simulink model "BatteryController_Rev1"  (Simulink 7.7)
settings: Solver=FixedStepDiscrete  StartTime=0.0  StopTime=10.0  RelTol=1e-3
PreLoadFcn:
  | try, eval([bdroot '_setup']); catch, eval('model_setup', ''); end
InitFcn:
  | try, eval([bdroot '_setup']); catch, eval('model_setup', ''); end
undefined symbols (not defined in the file or in its folder): ECU555, motohawk_build_version, motohawk_trunc_name, motohawk_vardec_path
libraries: MotoHawk_lib x213, motohawk_annotations_lib x6, motohawk_control_primitives_lib x2, simulink x1
(part 1 of 4)
Description:
  | Template Project Model
CloseFcn:
  | try, eval([bdroot '_close']); catch, eval('model_close', ''); end
settings Model: MotoHawkBuildVersion=073  MotoHawkBuildStats=struct('TotalFLASH',{0},'TotalEEPROM',{0},'TotalRAM',{0},'AppFLASH',{0},'AppEEPROM',{0},'AppRAM',{0},'HeapRAM',{0},'BuildSuccessCount',{73},'BuildErrorCount',{2})  MotoHawkModelSavedName=BatteryController_Rev1  MotoHawkModelGUID=1c823790-94c1-4f9f-95-ed-5c-78-f7-df-2e  MotoHawkModelOpenTime=2018 8 25 20 24 10.197  MotoHawkModelElapsedTime=15675530.773  MotoHawkBuildInfo=struct('model_name',{'BatteryController_Rev1'},'motohawk_version',{'2011a_sp0.184'},'motohawk_component_version',{'0.0.7'},'matlab_version',{'7.12.0'},'build_version',{'072'},'module_type',{'ECU555-48-0707'},'layout_type',{'PROD'},'processor_family',{'PPC'},'processor_type',{'MPC555'},'toolchain_vendor',{'gcc-powerpc-eabi'},'toolchain_version',{'4.4.0'},'component',{0},'archive_file',{'ECM.a'},'enable_build',{1},'fptype',{0},'flash_size',{368640},'ee_size',{4096},'ram_size',{26624},'decram_size',{0},'module_memory_def',{'MPC555_ModMemoryDef_4KEE_Prod'},'eri_table0_rev',{9},'max_eri_table_size',{65535},'use_debug_vardecs',{1},'use_info_vardecs',{1},'fgnd_base_period_ms',{5},'bgnd_base_period_ms',{50},'root_build_dir',{'C:\Users\maxar\Documents\GitHub\Wisconsin-Hybrid\BatteryController_Rev1'},'build_dir',{'C:\Users\maxar\Documents\GitHub\Wisconsin-Hybrid\BatteryController_Rev1\BatteryController_Rev1_Build'},'dll_name',{'BatteryCo_072'},'srz_name',{'BatteryController_Rev1_072'},'fgnd_stack_size',{3072},'fgnd_angle_stack_size',{0},'bgnd_stack_size',{2048},'idle_stack_size',{1024},'irq_stack_size',{1536},'heap_size',{4096},'heap_margin',{409},'install_dll_dir',{'C:\ECUFiles\TDBDLL\'},'install_srz_dir',{'C:\ECUFiles\Programs'},'app_int_stack_size',{1024},'shutdown_stack_size',{1024},'mingw_dir',{'C:\PROGRA~2\Woodward\DEVELO~1\TOOLCH~1\GCC\win32-pe\4_4_0\'},'motohawk_dir',{'C:\PROGRA~2\Woodward\MCS\MotoHawk\2011A_~1.184'},'toolchain_dir',{'C:\Program Files (x86)\Woodward\DevelopmentTools\Toolchains\GCC\powerpc-eabi\4_4_0\'},'matlab_root',{'C:\Program Files (x86)\MATLAB\R2011a'},'model_guid',{'1c823790-94c1-4f9f-95-ed-5c-78-f7-df-2e'},'build_guid',{'2c20b1f2-2f68-4f6b-8e-8e-5f-43-f8-60-40'},'token_guid',{'DD8AD11F95A6FC42BFF9AC780840E4B4'})  MotoHawkBuildGUID=2c20b1f2-2f68-4f6b-8e-8e-5f-43-f8-60-40  Creator=Owner  LastModifiedBy=maxar
settings OptimizationCC: InlineParams=on  InitFltsAndDblsToZero=on  OptimizeModelRefInitCode=on  LifeSpan=1
settings DebuggingCC: SolverPrmCheckMsg=none  InheritedTsInSrcMsg=none  TasksWithSamePriorityMsg=none  StrictBusMsg=Warning
settings HardwareCC: ProdEndianess=BigEndian  ProdHWDeviceType=Specified
settings RTWCC: SystemTargetFile=motohawk_ert_rtw.tlc  TLCOptions="-aCustomNonFinites=\"motohawk_genrtnonfinite.tlc\""  MakeCommand=motohawk_make_rtw  TemplateMakefile=motohawk_ert_rtw.tmf  Description=MotoHawk(tm) Rapid Prototyping  ProcessScript=motohawk_ert_rtw_make_rtw_hook
settings CodeAppCC: IgnoreCustomStorageClasses=off  MaxIdLength=100  CustomSymbolStrField=$H$N$M
settings STFCustomTargetCC: FunctionExecutionProfile=off  ModelReferenceCompliant=off  CombineOutputUpdateFcns=on  ERTCustomFileBanners=on  SupportContinuousTime=off  SupportNonInlinedSFcns=off  SystemTargetFile=motohawk_ert_rtw.tlc
settings ERTTargetCC: FunctionExecutionProfile=off  MultiwordLength=2048  ModelReferenceCompliant=off  ParMdlRefBuildCompliant=off  CompOptLevelCompliant=off  ERTFirstTimeCompliant=off  ModelStepFunctionPrototypeControlCompliant=off  CPPClassGenCompliant=off  ERTCustomFileTemplate=example_file_process.tlc  ConvertIfToSwitch=off

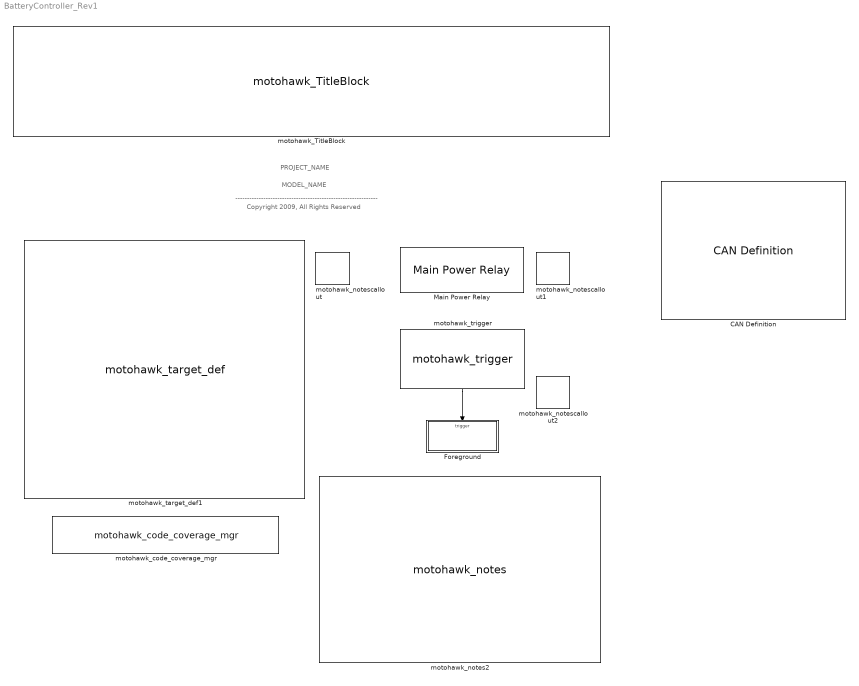
== system BatteryController_Rev1 ==
  note: PROJECT_NAME
  note: MODEL_NAME
  note: -------------------------------------------------------------
  note: Copyright 2009, All Rights Reserved
  CAN Definition : MotoHawk_lib/CAN Blocks/CAN Definition  Priority=-100  nam='CAN_1'  text_resource=CAN1  code_resource=NONE  val_resource=-1  target=ECU555-48-0707  bus=-2  btime=500 kbaud  pre=1  prop=0  pseg1=0  pseg2=0  resyn=0  tx_queue_size=16  rx_queue_size=16  use_protocol=on  city_id=hex2dec('D')  access_level=4  mototune_group='System | System Config | Communication Config'
  Foreground : Subsystem  TreatAsAtomicUnit=on
      mask init:
      | SampleTime = 0.005;
      | lbl = sprintf('%d ms', SampleTime * 1000);
      settings: RTWSystemCode=Function  RTWFcnNameOpts=Use subsystem name  RTWFileNameOpts=Use function name
      mask Display: disp(lbl);
  Main Power Relay : MotoHawk_lib/Extra Development Blocks/Main Power Relay  SystemSampleTime=-1  on_delay_count=2  off_delay_count=5  ecup_threshold=100  group='System | Main Power Relay'
  motohawk_TitleBlock : motohawk_annotations_lib/motohawk_TitleBlock  BlockType_='Mototron_Title_Block'  ttl="[  strrep(get_param(bdroot, 'Description') , '_', '\\_')  '\\newline\\rm'  'Top-level root of model:  '   strrep(bdroot, '_', '\\_') '.mdl'  ]"  copyright="'THE INFORMATION CONTAINED IN THIS\\newlineDRAWING IS THE SOLE PROPERTY OF\\newlineWOODWARD.  ANY REPRODUCTION IN\\newline PART OR AS A WHOLE WITHOUT THE\\newlineWRITTEN PERMISSION OF WOODWARD\\newline IS PROHIBITED.\\fontsize{16}\\rm\\copyright\\rm\\fontsize{10} 2009'"  address='\fontsize{22}\it\fontname{Arial Black}Woodward \fontname{Arial}\fontsize{10}\newline1000 East Drake Road, Fort Collins, CO, 80525\newlinemcs.woodward.com (866) 588-0494'  image_file='mh.jpg'  pretty_print=on  edit_text=|  edit_as=5
      | [
      | 
      | 
      | 
      | 
      | 
      | strrep(get_param(bdroot, 'Description') , '_', '\_')  '\newline\rm'
      | 
      | 
      | 
      | 
      | 
      | 'Top-level root of model:  '   strrep(bdroot, '_', '\_') '.mdl'
      | 
      | 
      | 
      | 
      | 
      | ]
  motohawk_code_coverage_mgr : MotoHawk_lib/Extra Development Blocks/motohawk_code_coverage_mgr  codegen=Always Generate Code Coverage Code  group='System | Code Coverage'
  motohawk_notes2 : motohawk_annotations_lib/motohawk_notes  BlockType_='Mototron_Notes'  desc="'\\fontname{wingdings 2}u\\fontname{arial}  The existence of a Target Definition block\\newlinesomewhere in the model sets it up as a\\newlineMotoHawk project, capable of being built to a\\newlineMotoTron target module.\\newline\\newline\\fontname{wingdings 2}v\\fontname{arial}  The Main Power Relay block monitors the\\newlinemodule power and controls the Main Power Relay\\newlineIt also performs startup and shutdown procedures\\newlinenecessary for EEPROM storage.  Most designs\\newlineshould contain this block\\newline\\newline\\fontname{wingdings 2}w\\fontname{arial}  All actions must be performed inside of a\\newlinefunction-call subsystem, triggered by a MotoHawk\\newlineentry-point trigger block, in order to be included in the\\newlinegenerated code.\\newline'"  edit_text=|  edit_as=2
      | \fontname{wingdings 2}u\fontname{arial}  The existence of a Target Definition block
      | 
      | 
      | somewhere in the model sets it up as a
      | 
      | 
      | MotoHawk project, capable of being built to a
      | 
      | 
      | Woodward target module.
      | 
      | 
      | 
      | 
      | 
      | \fontname{wingdings 2}v\fontname{arial}  The Main Power Relay block monitors the
      | 
      | 
      | module power and controls the Main Power Relay
      | 
      | 
      | It also performs startup and shutdown procedures
      | 
      | 
      | necessary for EEPROM storage.  Most designs
      | 
      | 
      | should contain this block
      | 
      | 
      | 
      | 
      | 
      | \fontname{wingdings 2}w\fontname{arial}  All actions must be performed inside of a
      | 
      | 
      | function-call subsystem, triggered by a MotoHawk
      | 
      | 
      | entry-point trigger block, in order to be included in the
      | 
      | 
      | generated code.
  motohawk_notescallout : motohawk_annotations_lib/motohawk_notescallout  BlockType_='Mototron_NoteCall'  desc='\bf1'
  motohawk_notescallout1 : motohawk_annotations_lib/motohawk_notescallout  BlockType_='Mototron_NoteCall'  desc='\bf2'
  motohawk_notescallout2 : motohawk_annotations_lib/motohawk_notescallout  BlockType_='Mototron_NoteCall'  desc='\bf3'
  motohawk_target_def1 : MotoHawk_lib/motohawk_target_def  Priority=-65535  target=ECU555-48-0707  layout=PROD  fptype=single (32 bits)  fgnd_stack_size=3*1024  fgnd_angle_stack_size=0  bgnd_stack_size=2*1024  idle_stack_size=1024  irq_stack_size=1536  app_int_stack_size=1024  shutdown_stack_size=1024  heap_size=4*1024  show_margins=off  fgnd_stack_margin=(3*1024) * 0.1  fgnd_angle_stack_margin=0  bgnd_stack_margin=(2*1024) * 0.1  idle_stack_margin=(1024) * 0.1  irq_stack_margin=(1536) * 0.1  app_int_stack_margin=(1024) * 0.1  shutdown_stack_margin=(1024) * 0.1  heap_margin=(4*1024) * 0.1  comp_name=bdroot  comp_img='KVASER_CAN_USB.jpg'  comp_security=No Encryption  comp_build_pass='mhbuild'  comp_sim_pass='mhsim'  comp_multi=off  show_filenames=off  dll_name=motohawk_trunc_name(bdroot, ['_' motohawk_build_version], 13)  srz_name=motohawk_trunc_name(bdroot, ['_' motohawk_build_version], 50)  build_dir='.'  comp_dir='.'
  motohawk_trigger : MotoHawk_lib/Trigger Blocks/motohawk_trigger  Tag=Trigger  Priority=0  trigger=FGND_RTI_PERIODIC  function_name=Trigger_FGND_RTI_PERIODIC_1023p0001  priority_order=0  inherited=off  run_disabled=off  override_app_monitor=off  target=ECU555_48_0707
  wires:
  motohawk_trigger/1 -> Foreground/Trigger

== system BatteryController_Rev1/Foreground ==
  f : TriggerPort  TriggerType=function-call
  Battery : Subsystem
  motohawk_TitleBlock : motohawk_annotations_lib/motohawk_TitleBlock  BlockType_='Mototron_Title_Block'  ttl=[strrep(get_param(bdroot, 'Description') , '_', '\_') '\newline\rm' get_param(gcs, 'Name')]  copyright="'THE INFORMATION CONTAINED IN THIS\\newlineDRAWING IS THE SOLE PROPERTY OF\\newlineWOODWARD.  ANY REPRODUCTION IN\\newline PART OR AS A WHOLE WITHOUT THE\\newlineWRITTEN PERMISSION OF WOODWARD\\newline IS PROHIBITED.\\fontsize{16}\\rm\\copyright\\rm\\fontsize{10} 2009'"  address='\fontsize{22}\it\fontname{Arial Black}Woodward \fontname{Arial}\fontsize{10}\newline1000 East Drake Road, Fort Collins, CO, 80525\newlinemcs.woodward.com (866) 588-0494'  image_file='mh.jpg'  pretty_print=on  edit_text=[strrep(get_param(bdroot, 'Description') , '_', '\_') '\newline\rm' get_param(gcs, 'Name')]  edit_as=5
  motohawk_code_coverage : MotoHawk_lib/Extra Development Blocks/motohawk_code_coverage

== system BatteryController_Rev1/Foreground/Battery ==
  Control : Subsystem
  Inputs : Subsystem
  Outputs : Subsystem
  wires:
  Control/1(Out1) -> Outputs/2(Controlled Inputs)
  Inputs/1(Out1) -> Control/1(In1), Outputs/1(Inputs)

== system BatteryController_Rev1/Foreground/Battery/Control ==
  In1 : Inport
  AMP Clamp : Subsystem
  Battery States : Subsystem
  Bus Creator : BusCreator  Inputs=3
  SOC : Subsystem
  Out1 : Outport
  wires:
  In1/1 -> Battery States/1(In1), SOC/1(In1), AMP Clamp/1(In1)
  Bus Creator/1 -> Out1/1
  Battery States/1(Out1) -> Bus Creator/1  "Battery States"
  AMP Clamp/1(Out1) -> Bus Creator/2, SOC/2(Current), Battery States/2(Current)  "AMP Clamp"
  SOC/1(Out1) -> Bus Creator/3  "SOC"

== system BatteryController_Rev1/Foreground/Battery/Inputs ==
  2G BMS : Subsystem
  AMP Clamp : Subsystem
  Bus Creator : BusCreator  Inputs=3
  Contactors : Subsystem
  Out1 : Outport
  wires:
  Bus Creator/1 -> Out1/1
  Contactors/1(Out1) -> Bus Creator/1  "Contactors"
  2G BMS/1(Out1) -> Bus Creator/2  "2G BMS"
  AMP Clamp/1(Out1) -> Bus Creator/3  "AMP Clamp"

== system BatteryController_Rev1/Foreground/Battery/Outputs ==
  Inputs : Inport
  Controlled Inputs : Inport  Port=2
  Battery : Subsystem
  Contactors : Subsystem
  wires:
  Controlled Inputs/1 -> Contactors/1(In1), Battery/2(Controlled Inputs)
  Inputs/1 -> Contactors/2(In2), Battery/1(Inputs)

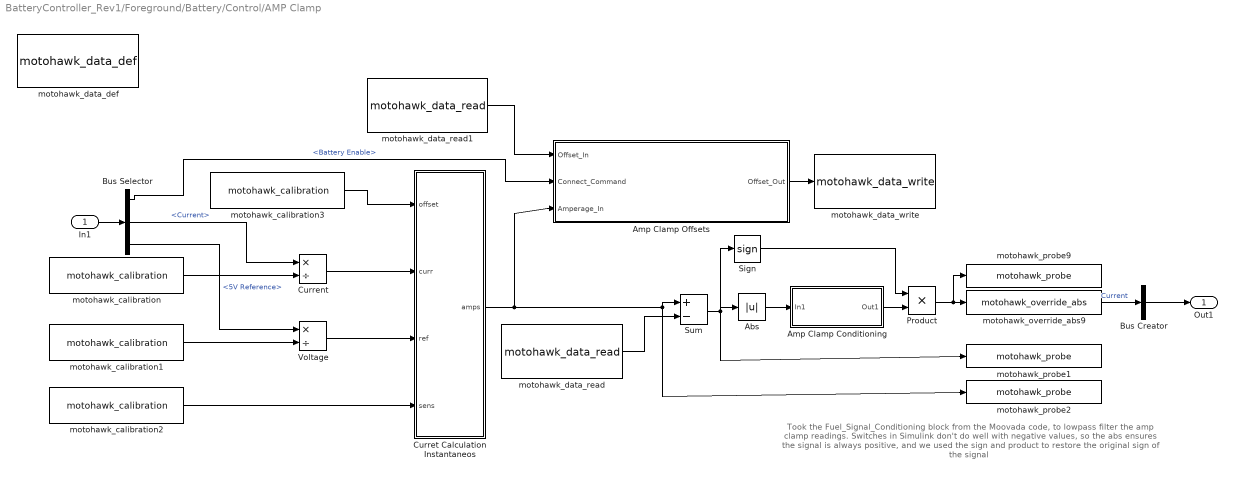
== system BatteryController_Rev1/Foreground/Battery/Control/AMP Clamp ==
  note: Took the Fuel_Signal_Conditioning block from the Moovada code, to lowpass filter the amp clamp readings.
      | Switches in Simulink don't do well with negative values, so the abs ensures the signal is always positive,
      | and we used the sign and product to restore the original sign of the signal
  In1 : Inport
  Abs : Abs
  Amp Clamp Conditioning : Subsystem
  Amp Clamp Offsets : Stateflow chart  TreatAsAtomicUnit=on
  Bus Creator : BusCreator  Inputs=1
  Bus Selector : BusSelector  OutputSignals=Contactors.Battery Enable,AMP Clamp.Current,AMP Clamp.5V Reference
  Current : Product  Inputs=*/  RndMeth=Zero
  Curret Calculation Instantaneos : Stateflow chart  TreatAsAtomicUnit=on
  Product : Product  RndMeth=Zero
  Sign : Signum
  Sum : Sum  Inputs=+-
  Voltage : Product  Inputs=*/  RndMeth=Zero
  motohawk_calibration : MotoHawk_lib/Calibration & Probing Blocks/motohawk_calibration  nam='Current_Div2'  val=819.2  storage=Calibration NV  show_more=off  name_source=Use Parameter  data_type=Inherit from 'Default Value'  read_level=1  write_level=1  ovr_cals=on  view_as=Number  enum_struct={'Disabled', 'Enabled'}  vector_style=Wide Row  use_help_units=off  help=''  units=''  use_header_enum=off  row_header_enum={}  col_header_enum={}  use_min_max=off  min_val=-inf  max_val=inf  use_precision=off  precision=''  gain=1  offset=0  exp=1  use_mototune_group=off  mototune_group=motohawk_vardec_path(gcb)
  motohawk_calibration1 : MotoHawk_lib/Calibration & Probing Blocks/motohawk_calibration  nam='V5V_Ref2'  val=409.6  storage=Calibration NV  show_more=off  name_source=Use Parameter  data_type=Inherit from 'Default Value'  read_level=1  write_level=1  ovr_cals=on  view_as=Number  enum_struct={'Disabled', 'Enabled'}  vector_style=Wide Row  use_help_units=off  help=''  units=''  use_header_enum=off  row_header_enum={}  col_header_enum={}  use_min_max=off  min_val=-inf  max_val=inf  use_precision=off  precision=''  gain=1  offset=0  exp=1  use_mototune_group=off  mototune_group=motohawk_vardec_path(gcb)
  motohawk_calibration2 : MotoHawk_lib/Calibration & Probing Blocks/motohawk_calibration  nam='G_Sensativity'  val=0.00615  storage=Calibration NV  show_more=on  name_source=Use Parameter  data_type=Inherit from 'Default Value'  read_level=1  write_level=1  ovr_cals=on  view_as=Number  enum_struct={'Disabled', 'Enabled'}  vector_style=Wide Row  use_help_units=on  help=''  units='V'  use_header_enum=off  row_header_enum={}  col_header_enum={}  use_min_max=off  min_val=-inf  max_val=inf  use_precision=on  precision='1.5'  gain=1  offset=0  exp=1  use_mototune_group=off  mototune_group=motohawk_vardec_path(gcb)
  motohawk_calibration3 : MotoHawk_lib/Calibration & Probing Blocks/motohawk_calibration  nam='AmpV_Offset'  val=2.15  storage=Calibration  show_more=off  name_source=Use Parameter  data_type=Inherit from 'Default Value'  read_level=1  write_level=1  ovr_cals=on  view_as=Number  enum_struct={'Disabled', 'Enabled'}  vector_style=Wide Row  use_help_units=off  help=''  units=''  use_header_enum=off  row_header_enum={}  col_header_enum={}  use_min_max=off  min_val=-inf  max_val=inf  use_precision=off  precision=''  gain=1  offset=0  exp=1  use_mototune_group=off  mototune_group=motohawk_vardec_path(gcb)
  motohawk_data_def : MotoHawk_lib/Data Storage Blocks/motohawk_data_def  nam='Amp_Offset'  container_nam=''  data=2.15  typ=double  struct_nam='MyStruct'  storage=NonVolatile  outputRef=off  use_vardec=on  window=Calibration  read_level=1  write_level=1  ovr_cals=on  view_as=Number  enum_struct={'Disabled', 'Enabled'}  vector_style=Wide Row  use_help_units=off  help=''  units=''  use_header_enum=off  row_header_enum=''  col_header_enum=''  use_min_max=off  min_val=-inf  max_val=inf  use_precision=off  precision=''  gain=1  offset=0  exp=1  use_mototune_group=off  mototune_group=motohawk_vardec_path(gcb)  eval_name=MyData  data_stores=motohawk_sfun_data_def_data_stores  struct_instances=motohawk_sfun_data_def_struct_instances  vardecs=motohawk_sfun_data_def_vardecs
  motohawk_data_read : MotoHawk_lib/Data Storage Blocks/motohawk_data_read  source=Lookup By Name  structure=Scalar  operation=Read scalar from location by index  sz_vec=4  sz_row=2  sz_col=3  typ=double  nam='Amp_Offset'  checkNull=on  struct_inst_name='MyData'  struct_nam='MyStruct'
  motohawk_data_read1 : MotoHawk_lib/Data Storage Blocks/motohawk_data_read  source=Lookup By Name  structure=Scalar  operation=Read scalar from location by index  sz_vec=4  sz_row=2  sz_col=3  typ=double  nam='Amp_Offset'  checkNull=on  struct_inst_name='MyData'  struct_nam='MyStruct'
  motohawk_data_write : MotoHawk_lib/Data Storage Blocks/motohawk_data_write  source=Lookup By Name  structure=Scalar  operation=Write entire data structure at once  sz_vec=9  sz_row=2  sz_col=9  typ=double  nam='Amp_Offset'  checkNull=on  write_read_only=off  struct_inst_name=''  struct_name='MyStruct'
  motohawk_override_abs9 : MotoHawk_lib/Calibration & Probing Blocks/motohawk_override_abs  SystemSampleTime=-1  parent_name='AMPCurrent_Ovr'  parent_val=0  show_more=on  name_source=Use Parameter  parent_read_level=1  parent_override_level=1  view_as=Number  enum_struct={'Disabled', 'Enabled'}  use_help_units=off  parent_help=''  parent_units=''  use_min_max=off  parent_min=-inf  parent_max=inf  use_precision=off  parent_precision=''  parent_gain=1  parent_offset=0  parent_exp=1  use_mototune_group=off  parent_group=motohawk_vardec_path(gcb)
  motohawk_probe1 : MotoHawk_lib/Calibration & Probing Blocks/motohawk_probe  nam='AMPCurrent_Pre_Filter_Prb'  show_more=on  name_source=Use Parameter  read_level=1  view_as=Number  enum_struct={'Disabled', 'Enabled'}  vector_style=Wide Row  use_help_units=on  help=''  units='A'  use_header_enum=off  row_header_enum={}  col_header_enum={}  use_precision=on  precision='1.5'  gain=1  offset=0  exp=1  use_mototune_group=off  mototune_group=motohawk_vardec_path(gcb)
  motohawk_probe2 : MotoHawk_lib/Calibration & Probing Blocks/motohawk_probe  nam='AMPCurrent_Pre_Offset_Prb'  show_more=on  name_source=Use Parameter  read_level=1  view_as=Number  enum_struct={'Disabled', 'Enabled'}  vector_style=Wide Row  use_help_units=on  help=''  units='A'  use_header_enum=off  row_header_enum={}  col_header_enum={}  use_precision=on  precision='1.5'  gain=1  offset=0  exp=1  use_mototune_group=off  mototune_group=motohawk_vardec_path(gcb)
  motohawk_probe9 : MotoHawk_lib/Calibration & Probing Blocks/motohawk_probe  nam='AMPCurrent_Prb'  show_more=on  name_source=Use Parameter  read_level=1  view_as=Number  enum_struct={'Disabled', 'Enabled'}  vector_style=Wide Row  use_help_units=on  help=''  units='A'  use_header_enum=off  row_header_enum={}  col_header_enum={}  use_precision=on  precision='1.5'  gain=1  offset=0  exp=1  use_mototune_group=off  mototune_group=motohawk_vardec_path(gcb)
  Out1 : Outport
  wires:
  In1/1 -> Bus Selector/1
  Bus Selector/2 -> Current/1  "<Current>"
  Bus Selector/3 -> Voltage/1  "<5V Reference>"
  Bus Creator/1 -> Out1/1
  motohawk_override_abs9/1 -> Bus Creator/1  "Current"
  motohawk_calibration1/1 -> Voltage/2
  motohawk_calibration/1 -> Current/2
  Current/1 -> Curret Calculation Instantaneos/2(curr)
  Voltage/1 -> Curret Calculation Instantaneos/3(ref)
  motohawk_calibration2/1 -> Curret Calculation Instantaneos/4(sens)
  Amp Clamp Conditioning/1(Out1) -> Product/2
  Sign/1 -> Product/1
  Product/1 -> motohawk_override_abs9/1, motohawk_probe9/1
  motohawk_calibration3/1 -> Curret Calculation Instantaneos/1(offset)
  Curret Calculation Instantaneos/1(amps) -> Amp Clamp Offsets/3(Amperage_In), Sum/1, motohawk_probe2/1
  Amp Clamp Offsets/1(Offset_Out) -> motohawk_data_write/1
  motohawk_data_read/1 -> Sum/2
  Sum/1 -> Abs/1, Sign/1, motohawk_probe1/1
  Abs/1 -> Amp Clamp Conditioning/1(In1)
  Bus Selector/1 -> Amp Clamp Offsets/2(Connect_Command)  "<Battery Enable>"
  motohawk_data_read1/1 -> Amp Clamp Offsets/1(Offset_In)

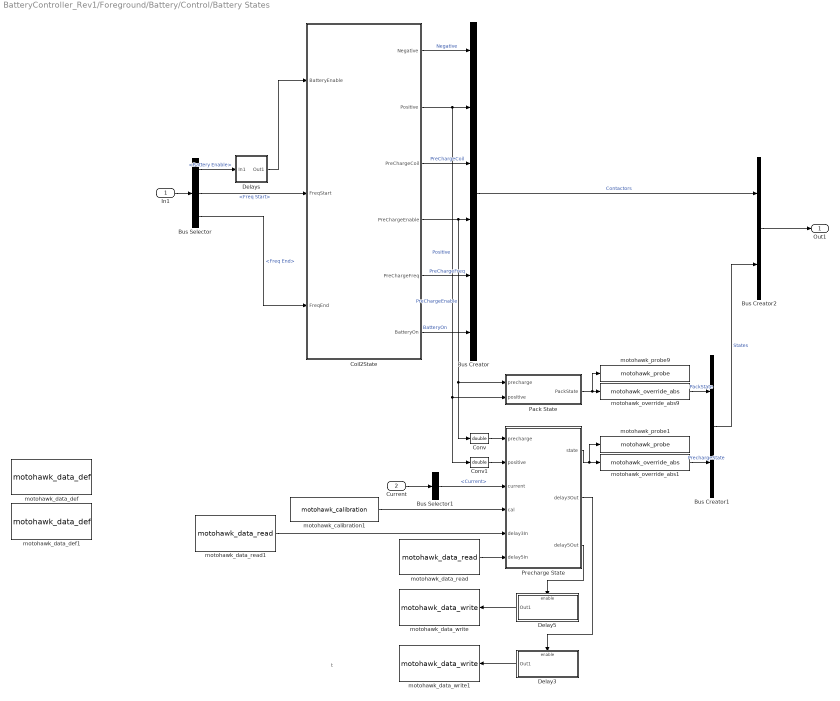
== system BatteryController_Rev1/Foreground/Battery/Control/Battery States ==
  note: t
  In1 : Inport
  Current : Inport  Port=2
  Bus Creator : BusCreator  Inputs=6
  Bus Creator1 : BusCreator  Inputs=2
  Bus Creator2 : BusCreator  Inputs=2
  Bus Selector : BusSelector  OutputSignals=Contactors.Battery Enable,Contactors.Freq Start,Contactors.Freq End
  Bus Selector1 : BusSelector  OutputSignals=Current
  Coil2State : Stateflow chart  TreatAsAtomicUnit=on
  Conv : DataTypeConversion  OutDataTypeStr=double
  Conv1 : DataTypeConversion  OutDataTypeStr=double
  Delay3 : Subsystem  TreatAsAtomicUnit=on
  Delay5 : Subsystem  TreatAsAtomicUnit=on
  Delays : Subsystem
  Pack State : Stateflow chart  TreatAsAtomicUnit=on
  Precharge State : Stateflow chart  TreatAsAtomicUnit=on
  motohawk_calibration1 : MotoHawk_lib/Calibration & Probing Blocks/motohawk_calibration  nam='Precharge_Current_Threshold'  val=.75  storage=Calibration NV  show_more=on  name_source=Use Parameter  data_type=Inherit from 'Default Value'  read_level=1  write_level=1  ovr_cals=on  view_as=Number  enum_struct={'Disabled', 'Enabled'}  vector_style=Wide Row  use_help_units=off  help=''  units=''  use_header_enum=off  row_header_enum={}  col_header_enum={}  use_min_max=off  min_val=-inf  max_val=inf  use_precision=off  precision=''  gain=1  offset=0  exp=1  use_mototune_group=off  mototune_group=motohawk_vardec_path(gcb)
  motohawk_data_def : MotoHawk_lib/Data Storage Blocks/motohawk_data_def  nam='Delay5'  container_nam=''  data=0  typ=boolean  struct_nam='MyStruct'  storage=Volatile  outputRef=off  use_vardec=on  window=Calibration  read_level=1  write_level=1  ovr_cals=on  view_as=Number  enum_struct={'Disabled', 'Enabled'}  vector_style=Wide Row  use_help_units=off  help=''  units=''  use_header_enum=off  row_header_enum=''  col_header_enum=''  use_min_max=off  min_val=-inf  max_val=inf  use_precision=off  precision=''  gain=1  offset=0  exp=1  use_mototune_group=off  mototune_group=motohawk_vardec_path(gcb)  eval_name=MyData  data_stores=motohawk_sfun_data_def_data_stores  struct_instances=motohawk_sfun_data_def_struct_instances  vardecs=motohawk_sfun_data_def_vardecs
  motohawk_data_def1 : MotoHawk_lib/Data Storage Blocks/motohawk_data_def  nam='Delay3'  container_nam=''  data=0  typ=boolean  struct_nam='MyStruct'  storage=Volatile  outputRef=off  use_vardec=on  window=Calibration  read_level=1  write_level=1  ovr_cals=on  view_as=Number  enum_struct={'Disabled', 'Enabled'}  vector_style=Wide Row  use_help_units=off  help=''  units=''  use_header_enum=off  row_header_enum=''  col_header_enum=''  use_min_max=off  min_val=-inf  max_val=inf  use_precision=off  precision=''  gain=1  offset=0  exp=1  use_mototune_group=off  mototune_group=motohawk_vardec_path(gcb)  eval_name=MyData  data_stores=motohawk_sfun_data_def_data_stores  struct_instances=motohawk_sfun_data_def_struct_instances  vardecs=motohawk_sfun_data_def_vardecs
  motohawk_data_read : MotoHawk_lib/Data Storage Blocks/motohawk_data_read  source=Lookup By Name  structure=Scalar  operation=Read scalar from location by index  sz_vec=4  sz_row=2  sz_col=3  typ=boolean  nam='Delay5'  checkNull=on  struct_inst_name='MyData'  struct_nam='MyStruct'
  motohawk_data_read1 : MotoHawk_lib/Data Storage Blocks/motohawk_data_read  source=Lookup By Name  structure=Scalar  operation=Read scalar from location by index  sz_vec=4  sz_row=2  sz_col=3  typ=boolean  nam='Delay3'  checkNull=on  struct_inst_name='MyData'  struct_nam='MyStruct'
  motohawk_data_write : MotoHawk_lib/Data Storage Blocks/motohawk_data_write  source=Lookup By Name  structure=Scalar  operation=Write entire data structure at once  sz_vec=9  sz_row=2  sz_col=9  typ=boolean  nam='Delay5'  checkNull=on  write_read_only=off  struct_inst_name=''  struct_name='MyStruct'
  motohawk_data_write1 : MotoHawk_lib/Data Storage Blocks/motohawk_data_write  source=Lookup By Name  structure=Scalar  operation=Write entire data structure at once  sz_vec=9  sz_row=2  sz_col=9  typ=boolean  nam='Delay3'  checkNull=on  write_read_only=off  struct_inst_name=''  struct_name='MyStruct'
  motohawk_override_abs1 : MotoHawk_lib/Calibration & Probing Blocks/motohawk_override_abs  SystemSampleTime=-1  parent_name='PrechargeState__Ovr'  parent_val=0  show_more=on  name_source=Use Parameter  parent_read_level=1  parent_override_level=1  view_as=Number  enum_struct={'Disabled', 'Enabled'}  use_help_units=off  parent_help=''  parent_units=''  use_min_max=off  parent_min=-inf  parent_max=inf  use_precision=off  parent_precision=''  parent_gain=1  parent_offset=0  parent_exp=1  use_mototune_group=off  parent_group=motohawk_vardec_path(gcb)
  motohawk_override_abs9 : MotoHawk_lib/Calibration & Probing Blocks/motohawk_override_abs  SystemSampleTime=-1  parent_name='PackState__Ovr'  parent_val=0  show_more=on  name_source=Use Parameter  parent_read_level=1  parent_override_level=1  view_as=Number  enum_struct={'Disabled', 'Enabled'}  use_help_units=off  parent_help=''  parent_units=''  use_min_max=off  parent_min=-inf  parent_max=inf  use_precision=off  parent_precision=''  parent_gain=1  parent_offset=0  parent_exp=1  use_mototune_group=off  parent_group=motohawk_vardec_path(gcb)
  motohawk_probe1 : MotoHawk_lib/Calibration & Probing Blocks/motohawk_probe  nam='PreChargeState__Prb'  show_more=on  name_source=Use Parameter  read_level=1  view_as=Number  enum_struct={'Disabled', 'Enabled'}  vector_style=Wide Row  use_help_units=off  help=''  units=''  use_header_enum=off  row_header_enum={}  col_header_enum={}  use_precision=off  precision=''  gain=1  offset=0  exp=1  use_mototune_group=off  mototune_group=motohawk_vardec_path(gcb)
  motohawk_probe9 : MotoHawk_lib/Calibration & Probing Blocks/motohawk_probe  nam='PackState__Prb'  show_more=on  name_source=Use Parameter  read_level=1  view_as=Number  enum_struct={'Disabled', 'Enabled'}  vector_style=Wide Row  use_help_units=off  help=''  units=''  use_header_enum=off  row_header_enum={}  col_header_enum={}  use_precision=off  precision=''  gain=1  offset=0  exp=1  use_mototune_group=off  mototune_group=motohawk_vardec_path(gcb)
  Out1 : Outport
  wires:
  In1/1 -> Bus Selector/1
  Bus Selector/2 -> Coil2State/2(FreqStart)  "<Freq Start>"
  Bus Selector/3 -> Coil2State/3(FreqEnd)  "<Freq End>"
  Coil2State/1(Negative) -> Bus Creator/1  "Negative"
  Coil2State/2(Positive) -> Bus Creator/2, Pack State/2(positive), Conv1/1  "Positive"
  Coil2State/3(PreChargeCoil) -> Bus Creator/3  "PreChargeCoil"
  Coil2State/4(PreChargeEnable) -> Bus Creator/4, Pack State/1(precharge), Conv/1  "PreChargeEnable"
  Coil2State/5(PreChargeFreq) -> Bus Creator/5  "PreChargeFreq"
  Coil2State/6(BatteryOn) -> Bus Creator/6  "BatteryOn"
  Current/1 -> Bus Selector1/1
  Bus Selector1/1 -> Precharge State/3(current)  "<Current>"
  motohawk_calibration1/1 -> Precharge State/4(cal)
  Bus Creator/1 -> Bus Creator2/1  "Contactors"
  Bus Creator2/1 -> Out1/1
  Bus Creator1/1 -> Bus Creator2/2  "States"
  Pack State/1(PackState) -> motohawk_override_abs9/1, motohawk_probe9/1
  motohawk_override_abs9/1 -> Bus Creator1/1  "PackState"
  Precharge State/1(state) -> motohawk_override_abs1/1, motohawk_probe1/1
  motohawk_override_abs1/1 -> Bus Creator1/2  "PrechargeState"
  Conv/1 -> Precharge State/1(precharge)
  Conv1/1 -> Precharge State/2(positive)
  Precharge State/2(delay3Out) -> Delay3/Enable
  Precharge State/3(delay5Out) -> Delay5/Enable
  motohawk_data_read/1 -> Precharge State/6(delay5In)
  Delay5/1(Out1) -> motohawk_data_write/1
  motohawk_data_read1/1 -> Precharge State/5(delay3In)
  Delay3/1(Out1) -> motohawk_data_write1/1
  Bus Selector/1 -> Delays/1(In1)  "<Battery Enable>"
  Delays/1(Out1) -> Coil2State/1(BatteryEnable)

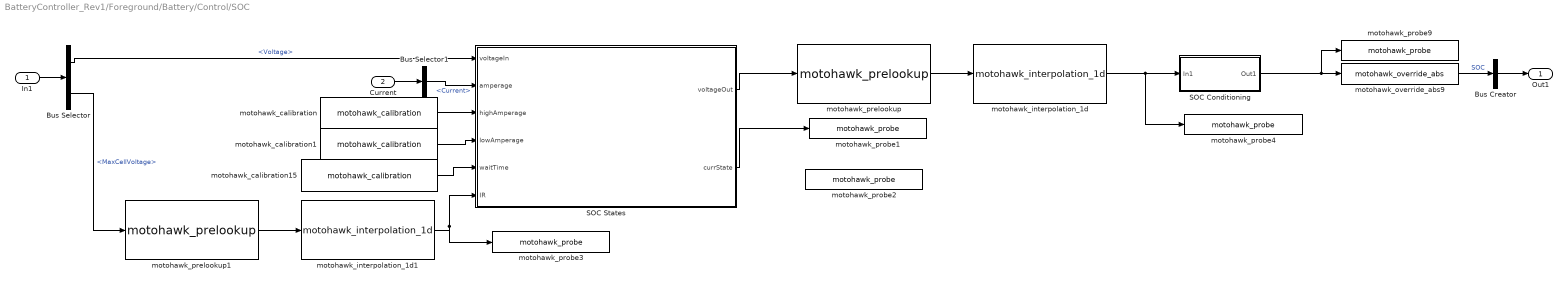
== system BatteryController_Rev1/Foreground/Battery/Control/SOC ==
  In1 : Inport
  Current : Inport  Port=2
  Bus Creator : BusCreator  Inputs=1
  Bus Selector : BusSelector  OutputSignals=2G BMS.Voltage,2G BMS.MaxCellVoltage
  Bus Selector1 : BusSelector  OutputSignals=Current
  SOC Conditioning : Subsystem
  SOC States : Stateflow chart  TreatAsAtomicUnit=on
  motohawk_calibration : MotoHawk_lib/Calibration & Probing Blocks/motohawk_calibration  nam='highAmperage'  val=25  storage=Calibration NV  show_more=on  name_source=Use Parameter  data_type=Inherit from 'Default Value'  read_level=1  write_level=1  ovr_cals=on  view_as=Number  enum_struct={'Disabled', 'Enabled'}  vector_style=Wide Row  use_help_units=off  help=''  units=''  use_header_enum=off  row_header_enum={}  col_header_enum={}  use_min_max=off  min_val=-inf  max_val=inf  use_precision=off  precision=''  gain=1  offset=0  exp=1  use_mototune_group=off  mototune_group=motohawk_vardec_path(gcb)
  motohawk_calibration1 : MotoHawk_lib/Calibration & Probing Blocks/motohawk_calibration  nam='lowAmperage'  val=20  storage=Calibration NV  show_more=on  name_source=Use Parameter  data_type=Inherit from 'Default Value'  read_level=1  write_level=1  ovr_cals=on  view_as=Number  enum_struct={'Disabled', 'Enabled'}  vector_style=Wide Row  use_help_units=on  help=''  units=''  use_header_enum=off  row_header_enum={}  col_header_enum={}  use_min_max=off  min_val=-inf  max_val=inf  use_precision=off  precision=''  gain=1  offset=0  exp=1  use_mototune_group=off  mototune_group=motohawk_vardec_path(gcb)
  motohawk_calibration15 : MotoHawk_lib/Calibration & Probing Blocks/motohawk_calibration  nam='Wait_time'  val=50  storage=Calibration NV  show_more=on  name_source=Use Parameter  data_type=int32  read_level=1  write_level=1  ovr_cals=on  view_as=Number  enum_struct={'Disabled', 'Enabled'}  vector_style=Wide Row  use_help_units=off  help=''  units=''  use_header_enum=off  row_header_enum={}  col_header_enum={}  use_min_max=off  min_val=-inf  max_val=inf  use_precision=on  precision=''  gain=0.05  offset=0  exp=1  use_mototune_group=off  mototune_group=motohawk_vardec_path(gcb)
  motohawk_interpolation_1d : MotoHawk_lib/Lookup Tables/motohawk_interpolation_1d  nam='SOCMap'  table_data=[100,99,8,0]  show_more=on  data_type=double  storage=Adaptive - NonVolatile  read_level=1  write_level=1  ovr_cals=on  use_help=off  help=''  units=''  use_min_max=on  min_val=0  max_val=100  use_precision=off  precision='1.2'  gain=1  offset=0  exp=1  use_links=on  prelookup_block='SOC_Table'  output_name=''  use_mototune_group=off  mototune_group=motohawk_vardec_path(gcb)
  motohawk_interpolation_1d1 : MotoHawk_lib/Lookup Tables/motohawk_interpolation_1d  nam='Temp_IR_Map'  table_data=[0.9,0.5,0.2,0.1,0.1]  show_more=on  data_type=double  storage=Adaptive - NonVolatile  read_level=1  write_level=1  ovr_cals=on  use_help=off  help=''  units=''  use_min_max=on  min_val=0  max_val=100  use_precision=off  precision='1.2'  gain=1  offset=0  exp=1  use_links=on  prelookup_block='Temp_IR_Table'  output_name=''  use_mototune_group=off  mototune_group=motohawk_vardec_path(gcb)
  motohawk_override_abs9 : MotoHawk_lib/Calibration & Probing Blocks/motohawk_override_abs  SystemSampleTime=-1  parent_name='SOC_Ovr'  parent_val=0  show_more=on  name_source=Use Parameter  parent_read_level=1  parent_override_level=1  view_as=Number  enum_struct={'Disabled', 'Enabled'}  use_help_units=off  parent_help=''  parent_units=''  use_min_max=off  parent_min=-inf  parent_max=inf  use_precision=off  parent_precision=''  parent_gain=1  parent_offset=0  parent_exp=1  use_mototune_group=off  parent_group=motohawk_vardec_path(gcb)
  motohawk_prelookup : MotoHawk_lib/Lookup Tables/motohawk_prelookup  nam='SOC_Table'  breakpoint_data=[385.95,378.51,319.92,279]  show_more=on  data_type=double  storage=NonVolatile  read_level=1  write_level=1  ovr_cals=on  use_help=off  help=''  units=''  use_min_max=off  min_val=-inf  max_val=inf  use_precision=off  precision=''  gain=1  offset=0  exp=1  use_links=off  input_name=''  use_mototune_group=off  mototune_group=motohawk_vardec_path(gcb)
  motohawk_prelookup1 : MotoHawk_lib/Lookup Tables/motohawk_prelookup  nam='Temp_IR_Table'  breakpoint_data=[-40,-20,0,20,40]  show_more=on  data_type=double  storage=NonVolatile  read_level=1  write_level=1  ovr_cals=on  use_help=off  help=''  units=''  use_min_max=off  min_val=-inf  max_val=inf  use_precision=off  precision=''  gain=1  offset=0  exp=1  use_links=off  input_name=''  use_mototune_group=off  mototune_group=motohawk_vardec_path(gcb)
  motohawk_probe1 : MotoHawk_lib/Calibration & Probing Blocks/motohawk_probe  nam='currState_Prb'  show_more=off  name_source=Use Parameter  read_level=1  view_as=Number  enum_struct={'Disabled', 'Enabled'}  vector_style=Wide Row  use_help_units=off  help=''  units=''  use_header_enum=off  row_header_enum={}  col_header_enum={}  use_precision=off  precision=''  gain=1  offset=0  exp=1  use_mototune_group=off  mototune_group=motohawk_vardec_path(gcb)
  motohawk_probe2 : MotoHawk_lib/Calibration & Probing Blocks/motohawk_probe  nam='vdiff_est_Prb'  show_more=off  name_source=Use Parameter  read_level=1  view_as=Number  enum_struct={'Disabled', 'Enabled'}  vector_style=Wide Row  use_help_units=off  help=''  units=''  use_header_enum=off  row_header_enum={}  col_header_enum={}  use_precision=off  precision=''  gain=1  offset=0  exp=1  use_mototune_group=off  mototune_group=motohawk_vardec_path(gcb)
  motohawk_probe3 : MotoHawk_lib/Calibration & Probing Blocks/motohawk_probe  nam='Temp_IR_Map_Prb'  show_more=off  name_source=Use Parameter  read_level=1  view_as=Number  enum_struct={'Disabled', 'Enabled'}  vector_style=Wide Row  use_help_units=off  help=''  units=''  use_header_enum=off  row_header_enum={}  col_header_enum={}  use_precision=off  precision=''  gain=1  offset=0  exp=1  use_mototune_group=off  mototune_group=motohawk_vardec_path(gcb)
  motohawk_probe4 : MotoHawk_lib/Calibration & Probing Blocks/motohawk_probe  nam='SOC_PreFilter_Prb'  show_more=off  name_source=Use Parameter  read_level=1  view_as=Number  enum_struct={'Disabled', 'Enabled'}  vector_style=Wide Row  use_help_units=off  help=''  units=''  use_header_enum=off  row_header_enum={}  col_header_enum={}  use_precision=off  precision=''  gain=1  offset=0  exp=1  use_mototune_group=off  mototune_group=motohawk_vardec_path(gcb)
  motohawk_probe9 : MotoHawk_lib/Calibration & Probing Blocks/motohawk_probe  nam='SOC_Prb'  show_more=on  name_source=Use Parameter  read_level=1  view_as=Number  enum_struct={'Disabled', 'Enabled'}  vector_style=Wide Row  use_help_units=off  help=''  units=''  use_header_enum=off  row_header_enum={}  col_header_enum={}  use_precision=off  precision=''  gain=1  offset=0  exp=1  use_mototune_group=off  mototune_group=motohawk_vardec_path(gcb)
  Out1 : Outport
  wires:
  In1/1 -> Bus Selector/1
  Bus Creator/1 -> Out1/1
  SOC States/1(voltageOut) -> motohawk_prelookup/1
  SOC States/2(currState) -> motohawk_probe1/1
  motohawk_calibration/1 -> SOC States/3(highAmperage)
  motohawk_calibration1/1 -> SOC States/4(lowAmperage)
  Current/1 -> Bus Selector1/1
  motohawk_override_abs9/1 -> Bus Creator/1  "SOC"
  motohawk_prelookup/1 -> motohawk_interpolation_1d/1
  motohawk_calibration15/1 -> SOC States/5(waitTime)
  ? -> motohawk_probe2/1
  Bus Selector/1 -> SOC States/1(voltageIn)  "<Voltage>"
  motohawk_prelookup1/1 -> motohawk_interpolation_1d1/1
  motohawk_interpolation_1d1/1 -> SOC States/6(IR), motohawk_probe3/1
  Bus Selector1/1 -> SOC States/2(amperage)  "<Current>"
  Bus Selector/2 -> motohawk_prelookup1/1  "<MaxCellVoltage>"
  motohawk_interpolation_1d/1 -> SOC Conditioning/1(In1), motohawk_probe4/1
  SOC Conditioning/1(Out1) -> motohawk_override_abs9/1, motohawk_probe9/1

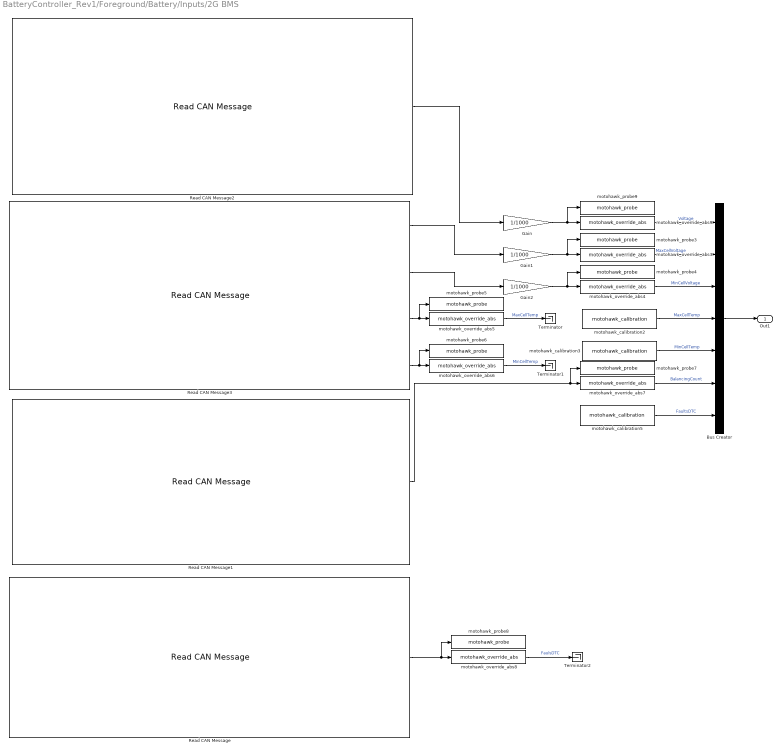
== system BatteryController_Rev1/Foreground/Battery/Inputs/2G BMS ==
  Bus Creator : BusCreator  Inputs=7
  Gain : Gain  Gain=1/1000
  Gain1 : Gain  Gain=1/1000
  Gain2 : Gain  Gain=1/1000
  Read CAN Message : MotoHawk_lib/CAN Blocks/Read CAN Message  nam='CAN_1'  bus=-2  msg=CANRx_VOLT_FAULTS  queue=1  slot=''  valid=off  stale=off  labelwires=off
  Read CAN Message1 : MotoHawk_lib/CAN Blocks/Read CAN Message  nam='CAN_1'  bus=-2  msg=CANRx_VOLT_SYSTEM_INFO  queue=1  slot=''  valid=off  stale=off  labelwires=off
  Read CAN Message2 : MotoHawk_lib/CAN Blocks/Read CAN Message  nam='CAN_1'  bus=-2  msg=CANRx_VOLT_PACK_V_I  queue=1  slot=''  valid=off  stale=off  labelwires=off
  Read CAN Message3 : MotoHawk_lib/CAN Blocks/Read CAN Message  nam='CAN_1'  bus=-2  msg=CANRx_VOLT_MINMAX_STATS  queue=1  slot=''  valid=off  stale=off  labelwires=off
  Terminator : Terminator
  Terminator1 : Terminator
  Terminator2 : Terminator
  motohawk_calibration2 : MotoHawk_lib/Calibration & Probing Blocks/motohawk_calibration  nam='MaxCellTemp'  val=25  storage=Calibration  show_more=off  name_source=Use Parameter  data_type=Inherit from 'Default Value'  read_level=1  write_level=1  ovr_cals=on  view_as=Number  enum_struct={'Disabled', 'Enabled'}  vector_style=Wide Row  use_help_units=off  help=''  units=''  use_header_enum=off  row_header_enum={}  col_header_enum={}  use_min_max=off  min_val=-inf  max_val=inf  use_precision=off  precision=''  gain=1  offset=0  exp=1  use_mototune_group=off  mototune_group=motohawk_vardec_path(gcb)
  motohawk_calibration3 : MotoHawk_lib/Calibration & Probing Blocks/motohawk_calibration  nam='MinCellTemp'  val=25  storage=Calibration  show_more=off  name_source=Use Parameter  data_type=Inherit from 'Default Value'  read_level=1  write_level=1  ovr_cals=on  view_as=Number  enum_struct={'Disabled', 'Enabled'}  vector_style=Wide Row  use_help_units=off  help=''  units=''  use_header_enum=off  row_header_enum={}  col_header_enum={}  use_min_max=off  min_val=-inf  max_val=inf  use_precision=off  precision=''  gain=1  offset=0  exp=1  use_mototune_group=off  mototune_group=motohawk_vardec_path(gcb)
  motohawk_calibration5 : MotoHawk_lib/Calibration & Probing Blocks/motohawk_calibration  nam='FaultsDTC'  val=0  storage=Calibration  show_more=off  name_source=Use Parameter  data_type=Inherit from 'Default Value'  read_level=1  write_level=1  ovr_cals=on  view_as=Number  enum_struct={'Disabled', 'Enabled'}  vector_style=Wide Row  use_help_units=off  help=''  units=''  use_header_enum=off  row_header_enum={}  col_header_enum={}  use_min_max=off  min_val=-inf  max_val=inf  use_precision=off  precision=''  gain=1  offset=0  exp=1  use_mototune_group=off  mototune_group=motohawk_vardec_path(gcb)
  motohawk_override_abs3 : MotoHawk_lib/Calibration & Probing Blocks/motohawk_override_abs  SystemSampleTime=-1  parent_name='MaxCellVoltage__Ovr'  parent_val=0  show_more=on  name_source=Use Parameter  parent_read_level=1  parent_override_level=1  view_as=Number  enum_struct={'Disabled', 'Enabled'}  use_help_units=off  parent_help=''  parent_units=''  use_min_max=off  parent_min=-inf  parent_max=inf  use_precision=off  parent_precision=''  parent_gain=1  parent_offset=0  parent_exp=1  use_mototune_group=off  parent_group=motohawk_vardec_path(gcb)
  motohawk_override_abs4 : MotoHawk_lib/Calibration & Probing Blocks/motohawk_override_abs  SystemSampleTime=-1  parent_name='MinCellVoltage__Ovr'  parent_val=0  show_more=on  name_source=Use Parameter  parent_read_level=1  parent_override_level=1  view_as=Number  enum_struct={'Disabled', 'Enabled'}  use_help_units=off  parent_help=''  parent_units=''  use_min_max=off  parent_min=-inf  parent_max=inf  use_precision=off  parent_precision=''  parent_gain=1  parent_offset=0  parent_exp=1  use_mototune_group=off  parent_group=motohawk_vardec_path(gcb)
  motohawk_override_abs5 : MotoHawk_lib/Calibration & Probing Blocks/motohawk_override_abs  SystemSampleTime=-1  parent_name='MaxCellTemp_Ovr'  parent_val=0  show_more=on  name_source=Use Parameter  parent_read_level=1  parent_override_level=1  view_as=Number  enum_struct={'Disabled', 'Enabled'}  use_help_units=off  parent_help=''  parent_units=''  use_min_max=off  parent_min=-inf  parent_max=inf  use_precision=off  parent_precision=''  parent_gain=1  parent_offset=0  parent_exp=1  use_mototune_group=off  parent_group=motohawk_vardec_path(gcb)
  motohawk_override_abs6 : MotoHawk_lib/Calibration & Probing Blocks/motohawk_override_abs  SystemSampleTime=-1  parent_name='MinCellTemp_Ovr'  parent_val=0  show_more=on  name_source=Use Parameter  parent_read_level=1  parent_override_level=1  view_as=Number  enum_struct={'Disabled', 'Enabled'}  use_help_units=off  parent_help=''  parent_units=''  use_min_max=off  parent_min=-inf  parent_max=inf  use_precision=off  parent_precision=''  parent_gain=1  parent_offset=0  parent_exp=1  use_mototune_group=off  parent_group=motohawk_vardec_path(gcb)
  motohawk_override_abs7 : MotoHawk_lib/Calibration & Probing Blocks/motohawk_override_abs  SystemSampleTime=-1  parent_name='BalancingCount_Ovr'  parent_val=0  show_more=on  name_source=Use Parameter  parent_read_level=1  parent_override_level=1  view_as=Number  enum_struct={'Disabled', 'Enabled'}  use_help_units=off  parent_help=''  parent_units=''  use_min_max=off  parent_min=-inf  parent_max=inf  use_precision=off  parent_precision=''  parent_gain=1  parent_offset=0  parent_exp=1  use_mototune_group=off  parent_group=motohawk_vardec_path(gcb)
  motohawk_override_abs8 : MotoHawk_lib/Calibration & Probing Blocks/motohawk_override_abs  SystemSampleTime=-1  parent_name='FaultsDTC_Ovr'  parent_val=0  show_more=on  name_source=Use Parameter  parent_read_level=1  parent_override_level=1  view_as=Number  enum_struct={'Disabled', 'Enabled'}  use_help_units=off  parent_help=''  parent_units=''  use_min_max=off  parent_min=-inf  parent_max=inf  use_precision=off  parent_precision=''  parent_gain=1  parent_offset=0  parent_exp=1  use_mototune_group=off  parent_group=motohawk_vardec_path(gcb)
  motohawk_override_abs9 : MotoHawk_lib/Calibration & Probing Blocks/motohawk_override_abs  SystemSampleTime=-1  parent_name='Voltage_Ovr'  parent_val=0  show_more=on  name_source=Use Parameter  parent_read_level=1  parent_override_level=1  view_as=Number  enum_struct={'Disabled', 'Enabled'}  use_help_units=off  parent_help=''  parent_units=''  use_min_max=off  parent_min=-inf  parent_max=inf  use_precision=off  parent_precision=''  parent_gain=1  parent_offset=0  parent_exp=1  use_mototune_group=off  parent_group=motohawk_vardec_path(gcb)
  motohawk_probe3 : MotoHawk_lib/Calibration & Probing Blocks/motohawk_probe  nam='MaxCellVoltage__Prb'  show_more=on  name_source=Use Parameter  read_level=1  view_as=Number  enum_struct={'Disabled', 'Enabled'}  vector_style=Wide Row  use_help_units=off  help=''  units=''  use_header_enum=off  row_header_enum={}  col_header_enum={}  use_precision=off  precision=''  gain=1  offset=0  exp=1  use_mototune_group=off  mototune_group=motohawk_vardec_path(gcb)
  motohawk_probe4 : MotoHawk_lib/Calibration & Probing Blocks/motohawk_probe  nam='MinCellVoltage__Prb'  show_more=on  name_source=Use Parameter  read_level=1  view_as=Number  enum_struct={'Disabled', 'Enabled'}  vector_style=Wide Row  use_help_units=off  help=''  units=''  use_header_enum=off  row_header_enum={}  col_header_enum={}  use_precision=off  precision=''  gain=1  offset=0  exp=1  use_mototune_group=off  mototune_group=motohawk_vardec_path(gcb)
  motohawk_probe5 : MotoHawk_lib/Calibration & Probing Blocks/motohawk_probe  nam='MaxCellTemp_Prb'  show_more=on  name_source=Use Parameter  read_level=1  view_as=Number  enum_struct={'Disabled', 'Enabled'}  vector_style=Wide Row  use_help_units=off  help=''  units=''  use_header_enum=off  row_header_enum={}  col_header_enum={}  use_precision=off  precision=''  gain=1  offset=0  exp=1  use_mototune_group=off  mototune_group=motohawk_vardec_path(gcb)
  motohawk_probe6 : MotoHawk_lib/Calibration & Probing Blocks/motohawk_probe  nam='MinCellTemp_Prb'  show_more=on  name_source=Use Parameter  read_level=1  view_as=Number  enum_struct={'Disabled', 'Enabled'}  vector_style=Wide Row  use_help_units=off  help=''  units=''  use_header_enum=off  row_header_enum={}  col_header_enum={}  use_precision=off  precision=''  gain=1  offset=0  exp=1  use_mototune_group=off  mototune_group=motohawk_vardec_path(gcb)
  motohawk_probe7 : MotoHawk_lib/Calibration & Probing Blocks/motohawk_probe  nam='BalancingCount_Prb'  show_more=on  name_source=Use Parameter  read_level=1  view_as=Number  enum_struct={'Disabled', 'Enabled'}  vector_style=Wide Row  use_help_units=off  help=''  units=''  use_header_enum=off  row_header_enum={}  col_header_enum={}  use_precision=off  precision=''  gain=1  offset=0  exp=1  use_mototune_group=off  mototune_group=motohawk_vardec_path(gcb)
  motohawk_probe8 : MotoHawk_lib/Calibration & Probing Blocks/motohawk_probe  nam='FaultsDTC_Prb'  show_more=on  name_source=Use Parameter  read_level=1  view_as=Number  enum_struct={'Disabled', 'Enabled'}  vector_style=Wide Row  use_help_units=off  help=''  units=''  use_header_enum=off  row_header_enum={}  col_header_enum={}  use_precision=off  precision=''  gain=1  offset=0  exp=1  use_mototune_group=off  mototune_group=motohawk_vardec_path(gcb)
  motohawk_probe9 : MotoHawk_lib/Calibration & Probing Blocks/motohawk_probe  nam='Voltage_Prb'  show_more=on  name_source=Use Parameter  read_level=1  view_as=Number  enum_struct={'Disabled', 'Enabled'}  vector_style=Wide Row  use_help_units=off  help=''  units=''  use_header_enum=off  row_header_enum={}  col_header_enum={}  use_precision=off  precision=''  gain=1  offset=0  exp=1  use_mototune_group=off  mototune_group=motohawk_vardec_path(gcb)
  Out1 : Outport
  wires:
  Bus Creator/1 -> Out1/1
  motohawk_override_abs9/1 -> Bus Creator/1  "Voltage"
  Read CAN Message2/1 -> Gain/1
  motohawk_override_abs3/1 -> Bus Creator/2  "MaxCellVoltage"
  motohawk_override_abs4/1 -> Bus Creator/3  "MinCellVoltage"
  motohawk_override_abs7/1 -> Bus Creator/6  "BalancingCount"
  Gain/1 -> motohawk_override_abs9/1, motohawk_probe9/1
  Gain1/1 -> motohawk_override_abs3/1, motohawk_probe3/1
  Gain2/1 -> motohawk_override_abs4/1, motohawk_probe4/1
  Read CAN Message1/1 -> motohawk_override_abs7/1, motohawk_probe7/1
  Read CAN Message3/1 -> Gain1/1
  Read CAN Message3/2 -> Gain2/1
  motohawk_calibration2/1 -> Bus Creator/4  "MaxCellTemp"
  motohawk_calibration3/1 -> Bus Creator/5  "MinCellTemp"
  Read CAN Message3/3 -> motohawk_override_abs5/1, motohawk_probe5/1
  Read CAN Message3/4 -> motohawk_override_abs6/1, motohawk_probe6/1
  motohawk_override_abs5/1 -> Terminator/1  "MaxCellTemp"
  motohawk_override_abs6/1 -> Terminator1/1  "MinCellTemp"
  motohawk_calibration5/1 -> Bus Creator/7  "FaultsDTC"
  Read CAN Message/1 -> motohawk_override_abs8/1, motohawk_probe8/1
  motohawk_override_abs8/1 -> Terminator2/1  "FaulsDTC"
